simulink model "faren"  (Simulink 7.6)
settings: Solver=ode4  StartTime=0.0  StopTime=inf  FixedStep=0.5  RelTol=1e-3
undefined symbols (not defined in the file or in its folder): bit, Standard
libraries: xpclib x9, simulink x2
settings Model: xpc_rtwmakecfg_data=_xpccanac2pci_  Creator=Administrator  LastModifiedBy=Administrator  SimulationMode=external  BufferReuse=off
settings OptimizationCC: BlockReduction=off  OptimizeBlockIOStorage=off  BufferReuse=off  ExpressionFolding=off  LocalBlockOutputs=off
settings HardwareCC: ProdIntDivRoundTo=Zero  ProdEndianess=LittleEndian  ProdHWDeviceType=Generic->32-bit x86 compatible
settings RTWCC: SystemTargetFile=xpctarget.tlc  TemplateMakefile=xpc_default_tmf  Description=xPC Target  ProcessScript=xpctarget_make_rtw_hook  RTWCompilerOptimization=On
settings xpcTargetCC: TargetFcnLib=ansi_tfl_table_tmw.mat  TargetFunctionLibrary=XPC_BLAS  ERTCodeCoverageTool=None  ParMdlRefBuildCompliant=on  CombineSignalStateStructs=off  PortableWordSizes=off  xPCLoadParamSetFile=off  xPCConcurrentTasks=off  xPCEnableSFAnimation=off

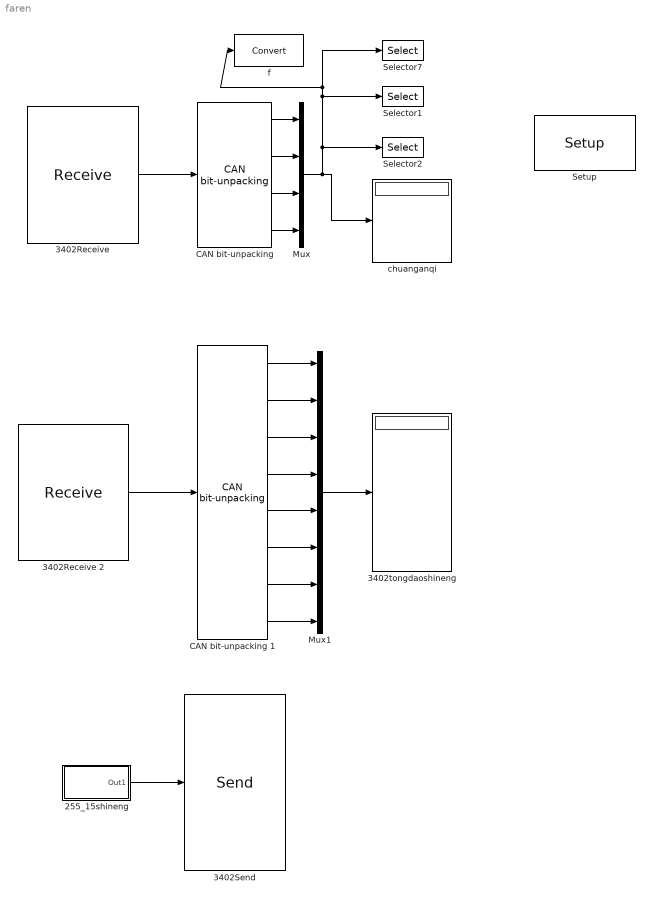
== system faren ==
  255_15shineng : Subsystem
  "3402Receive " : xpclib/CAN/Softing/CAN-AC2-PCI SJA 1000/Receive   board=1  canPort=CAN 2  range=Standard (11-bit)  ids=[386]  lengths=0  output=Data  inten=off  ts=-1  ididx=[0]
  3402Receive 2 : xpclib/CAN/Softing/CAN-AC2-PCI SJA 1000/Receive   board=1  canPort=CAN 2  range=Standard (11-bit)  ids=1410  lengths=0  output=Data  inten=off  ts=-1  ididx=[1]
  3402Send : xpclib/CAN/Softing/CAN-AC2-PCI SJA 1000/Send   board=1  canPort=CAN 2  range=Standard (11-bit)  ids=[1538]  sizes=[8]  output=off  ts=-1  ididx=[0]
  3402tongdaoshineng : Display
  "CAN bit-unpacking " : xpclib/CAN/Utilities/CAN bit-unpacking   bitpatterns={ [0:15],[16:31],[32:47],[48:63] }  dtypes={ 'uint16','uint16','uint16','uint16' }
  CAN bit-unpacking 1 : xpclib/CAN/Utilities/CAN bit-unpacking   bitpatterns={ [0:7],[8:15],[16:23],[24:31],[32:39],[40:47],[48:55],[56:63] }  dtypes={ 'uint8','uint8','uint8','uint8','uint8','uint8','uint8','uint8' }
  Mux : Mux
  Mux1 : Mux  Inputs=8
  Selector1 : Selector  IndexOptions=Index vector (dialog)  Indices=2  OutputSizes=1
  Selector2 : Selector  IndexOptions=Index vector (dialog)  Indices=3  OutputSizes=1
  Selector7 : Selector  IndexOptions=Index vector (dialog)  Indices=1  OutputSizes=1
  "Setup " : xpclib/CAN/Softing/CAN-AC2-PCI SJA 1000/Setup   board=1  can1bus=Lowspeed (requires LS module)  can1Baudrate=10 kBaud  can1UserBR=[1,1,4,3]  can2bus=Lowspeed (requires LS module)  can2Baudrate=10 kBaud  can2UserBR=[1,1,4,3]  init=[]  term=[]  bus_off_out=off  bus_off_rec=Off  ioBaseAddress=-1
  chuanganqi : Display
  f : DataTypeConversion
  wires:
  255_15shineng/1(Out1) -> 3402Send/1
  "3402Receive "/1 -> "CAN bit-unpacking "/1
  "CAN bit-unpacking "/1 -> Mux/1
  "CAN bit-unpacking "/2 -> Mux/2
  "CAN bit-unpacking "/3 -> Mux/3
  "CAN bit-unpacking "/4 -> Mux/4
  CAN bit-unpacking 1/1 -> Mux1/1
  CAN bit-unpacking 1/2 -> Mux1/2
  CAN bit-unpacking 1/3 -> Mux1/3
  CAN bit-unpacking 1/4 -> Mux1/4
  CAN bit-unpacking 1/5 -> Mux1/5
  CAN bit-unpacking 1/6 -> Mux1/6
  CAN bit-unpacking 1/7 -> Mux1/7
  CAN bit-unpacking 1/8 -> Mux1/8
  3402Receive 2/1 -> CAN bit-unpacking 1/1
  Mux1/1 -> 3402tongdaoshineng/1
  Mux/1 -> chuanganqi/1, Selector7/1, f/1, Selector1/1, Selector2/1

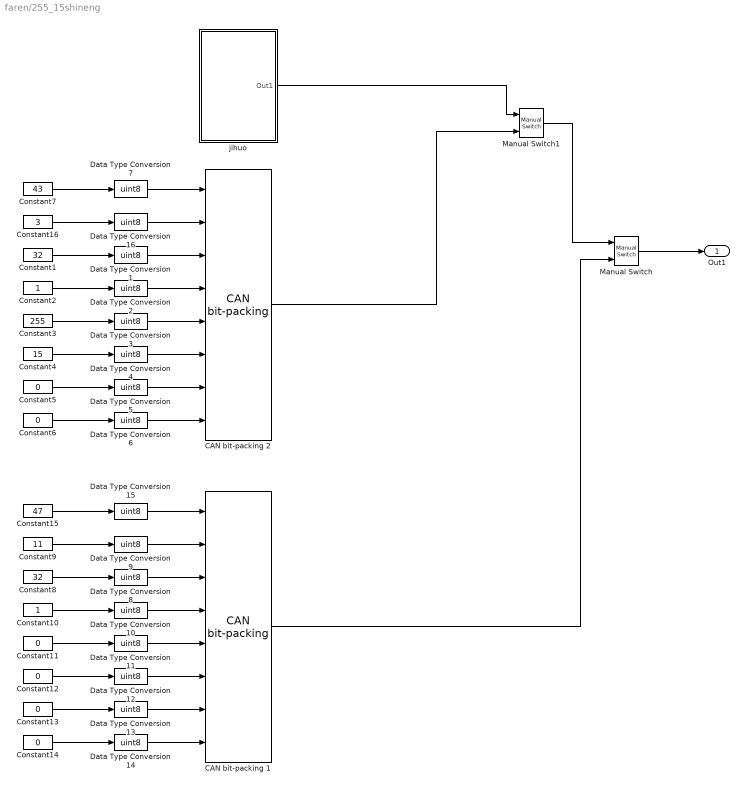
== system faren/255_15shineng ==
  CAN bit-packing 1 : xpclib/CAN/Utilities/CAN bit-packing   bitpatterns={ [0:7],[8:15],[16:23],[24:31],[32:39],[40:47],[48:55],[56:63] }
  CAN bit-packing 2 : xpclib/CAN/Utilities/CAN bit-packing   bitpatterns={ [0:7],[8:15],[16:23],[24:31],[32:39],[40:47],[48:55],[56:63] }
  Constant1 : Constant  Value=32
  Constant10 : Constant
  Constant{5..6,11..14} (6 alike) : Constant  Value=0
  Constant15 : Constant  Value=47
  Constant16 : Constant  Value=3
  Constant2 : Constant
  Constant3 : Constant  Value=255
  Constant4 : Constant  Value=15
  Constant7 : Constant  Value=43
  Constant8 : Constant  Value=32
  Constant9 : Constant  Value=11
  Data Type Conversion{1..16} (16 alike) : DataTypeConversion  OutDataTypeStr=uint8
  Manual Switch : simulink/Signal Routing/Manual Switch  SystemSampleTime=-1  sw=1  action=0  varsize=off
  Manual Switch1 : simulink/Signal Routing/Manual Switch  SystemSampleTime=-1  sw=1  action=0  varsize=off
  jihuo : Subsystem
  Out1 : Outport
  wires:
  Data Type Conversion7/1 -> CAN bit-packing 2/1
  Data Type Conversion16/1 -> CAN bit-packing 2/2
  Data Type Conversion1/1 -> CAN bit-packing 2/3
  Data Type Conversion2/1 -> CAN bit-packing 2/4
  Data Type Conversion3/1 -> CAN bit-packing 2/5
  Data Type Conversion4/1 -> CAN bit-packing 2/6
  Data Type Conversion5/1 -> CAN bit-packing 2/7
  Data Type Conversion6/1 -> CAN bit-packing 2/8
  Constant7/1 -> Data Type Conversion7/1
  Constant16/1 -> Data Type Conversion16/1
  Constant1/1 -> Data Type Conversion1/1
  Constant2/1 -> Data Type Conversion2/1
  Constant3/1 -> Data Type Conversion3/1
  Constant4/1 -> Data Type Conversion4/1
  Constant5/1 -> Data Type Conversion5/1
  Constant6/1 -> Data Type Conversion6/1
  Data Type Conversion15/1 -> CAN bit-packing 1/1
  Data Type Conversion9/1 -> CAN bit-packing 1/2
  Data Type Conversion8/1 -> CAN bit-packing 1/3
  Data Type Conversion10/1 -> CAN bit-packing 1/4
  Data Type Conversion11/1 -> CAN bit-packing 1/5
  Data Type Conversion12/1 -> CAN bit-packing 1/6
  Data Type Conversion13/1 -> CAN bit-packing 1/7
  Data Type Conversion14/1 -> CAN bit-packing 1/8
  Constant15/1 -> Data Type Conversion15/1
  Constant9/1 -> Data Type Conversion9/1
  Constant8/1 -> Data Type Conversion8/1
  Constant10/1 -> Data Type Conversion10/1
  Constant11/1 -> Data Type Conversion11/1
  Constant12/1 -> Data Type Conversion12/1
  Constant13/1 -> Data Type Conversion13/1
  Constant14/1 -> Data Type Conversion14/1
  CAN bit-packing 1/1 -> Manual Switch/2
  CAN bit-packing 2/1 -> Manual Switch1/2
  Manual Switch/1 -> Out1/1
  jihuo/1(Out1) -> Manual Switch1/1
  Manual Switch1/1 -> Manual Switch/1

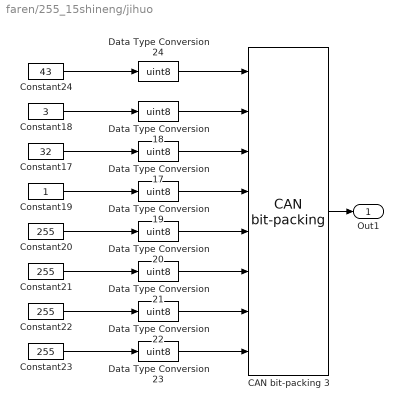
== system faren/255_15shineng/jihuo ==
  CAN bit-packing 3 : xpclib/CAN/Utilities/CAN bit-packing   bitpatterns={ [0:7],[8:15],[16:23],[24:31],[32:39],[40:47],[48:55],[56:63] }
  Constant17 : Constant  Value=32
  Constant18 : Constant  Value=3
  Constant19 : Constant
  Constant{20..23} (4 alike) : Constant  Value=255
  Constant24 : Constant  Value=43
  Data Type Conversion{17..24} (8 alike) : DataTypeConversion  OutDataTypeStr=uint8
  Out1 : Outport
  wires:
  Data Type Conversion24/1 -> CAN bit-packing 3/1
  Data Type Conversion18/1 -> CAN bit-packing 3/2
  Data Type Conversion17/1 -> CAN bit-packing 3/3
  Data Type Conversion19/1 -> CAN bit-packing 3/4
  Data Type Conversion20/1 -> CAN bit-packing 3/5
  Data Type Conversion21/1 -> CAN bit-packing 3/6
  Data Type Conversion22/1 -> CAN bit-packing 3/7
  Data Type Conversion23/1 -> CAN bit-packing 3/8
  Constant24/1 -> Data Type Conversion24/1
  Constant18/1 -> Data Type Conversion18/1
  Constant17/1 -> Data Type Conversion17/1
  Constant19/1 -> Data Type Conversion19/1
  Constant20/1 -> Data Type Conversion20/1
  Constant21/1 -> Data Type Conversion21/1
  Constant22/1 -> Data Type Conversion22/1
  Constant23/1 -> Data Type Conversion23/1
  CAN bit-packing 3/1 -> Out1/1
